simulink model "LQR_EXwithPI"  (Simulink 7.9)
settings: Solver=ode45  StartTime=0.0  StopTime=5  MaxStep=1e-3  RelTol=1e-3
values from neighbouring files (symbols this model uses):
  K1 = K(1,1)    [file_for_LQR_EX.m]
  K2 = K(1,2)    [file_for_LQR_EX.m]
  Q = [2 1; 1 4]    [Riccati_sol2.m]    (also in file_for_LQR_EX.m = [100 0 ; 0 0]; inf_horiz.m = [10 0; 0 2000])
  R = 1/2    (= 0.5)    [Riccati_sol2.m]    (also in file_for_LQR_EX.m = 10; inf_horiz.m = 1)
libraries: simulink x1
settings Model: Creator=DR_C  LastModifiedBy=DR_C
settings DataIOCC: SignalLoggingName=sigsOut
settings OptimizationCC: InitFltsAndDblsToZero=on
settings DebuggingCC: SaveWithParameterizedLinksMsg=none  SignalResolutionControl=TryResolveAllWithWarning  SolverPrmCheckMsg=none  MultiTaskDSMMsg=warning  MultiTaskCondExecSysMsg=none  FcnCallInpInsideContextMsg=Use local settings  StrictBusMsg=Warning
settings HardwareCC: TargetUnknown=on
settings RTWCC: IncludeERTFirstTime=on
settings GRTTargetCC: TargetFcnLib=ansi_tfl_tmw.mat  CombineOutputUpdateFcns=off  GRTInterface=on

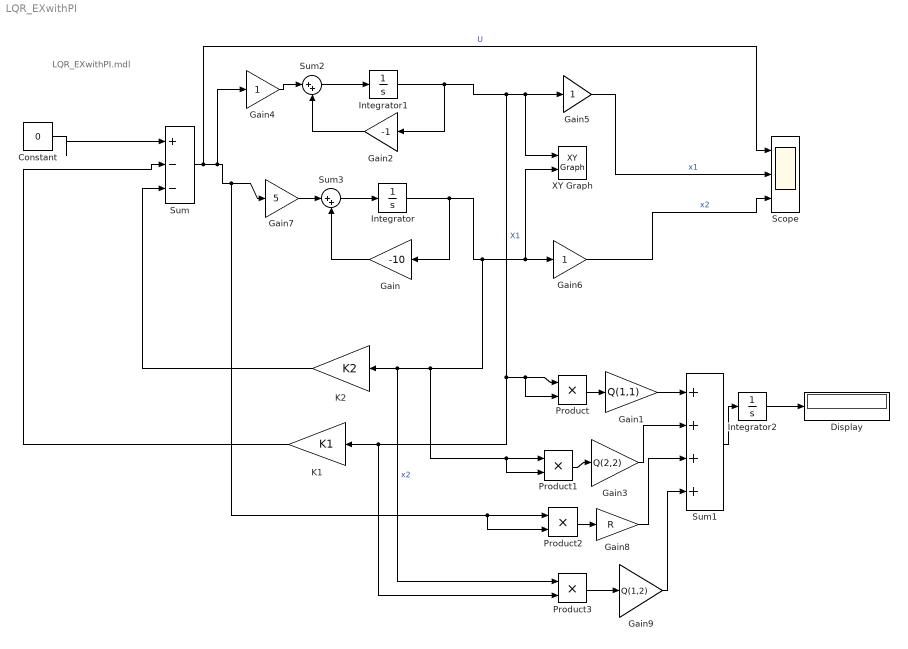
== system LQR_EXwithPI ==
  note: LQR_EXwithPI.mdl
  Constant : Constant  Value=0
  Display : Display
  Gain : Gain  Gain=-10  SaturateOnIntegerOverflow=on  OutDataTypeStr=Inherit: Same as input  ParamDataTypeStr=Inherit: Same as input
  Gain1 : Gain  Gain=Q(1,1)
  Gain2 : Gain  Gain=-1  SaturateOnIntegerOverflow=on  OutDataTypeStr=Inherit: Same as input  ParamDataTypeStr=Inherit: Same as input
  Gain3 : Gain  Gain=Q(2,2)
  Gain4 : Gain  SaturateOnIntegerOverflow=on  OutDataTypeStr=Inherit: Same as input  ParamDataTypeStr=Inherit: Same as input
  Gain5 : Gain  SaturateOnIntegerOverflow=on  OutDataTypeStr=Inherit: Same as input  ParamDataTypeStr=Inherit: Same as input
  Gain6 : Gain  SaturateOnIntegerOverflow=on  OutDataTypeStr=Inherit: Same as input  ParamDataTypeStr=Inherit: Same as input
  Gain7 : Gain  Gain=5  SaturateOnIntegerOverflow=on  OutDataTypeStr=Inherit: Same as input  ParamDataTypeStr=Inherit: Same as input
  Gain8 : Gain  Gain=R
  Gain9 : Gain  Gain=Q(1,2)
  Integrator : Integrator  InitialCondition=10
  Integrator1 : Integrator  InitialCondition=10
  Integrator2 : Integrator
  K1 : Gain  Gain=K1  SaturateOnIntegerOverflow=on  OutDataTypeStr=Inherit: Same as input  ParamDataTypeStr=Inherit: Same as input
  K2 : Gain  Gain=K2  SaturateOnIntegerOverflow=on  OutDataTypeStr=Inherit: Same as input  ParamDataTypeStr=Inherit: Same as input
  Product{,1..3} (4 alike) : Product  RndMeth=Zero
  Scope : Scope  NumInputPorts=3
      settings: YMin=-0.009~0~-0.007  YMax=0~0.004~0
  Sum : Sum  Inputs=|+--  SaturateOnIntegerOverflow=on
  Sum1 : Sum  Inputs=++++
  Sum2 : Sum  Inputs=|++  SaturateOnIntegerOverflow=on
  Sum3 : Sum  Inputs=|++  SaturateOnIntegerOverflow=on
  XY Graph : simulink/Sinks/XY Graph  xmin=-10  xmax=10  ymin=-10  ymax=10  st=-1
  wires:
  Gain5/1 -> Scope/2  "x1"
  Gain6/1 -> Scope/3  "x2"
  Integrator1/1 -> Gain2/1, Gain5/1, XY Graph/1, Product/1, Product/2, K1/1, Product3/2  "X1"
  Integrator/1 -> Gain/1, Gain6/1, XY Graph/2, Product1/1, Product1/2, K2/1, Product3/1  "x2"
  Sum/1 -> Gain4/1, Gain7/1, Product2/1, Product2/2, Scope/1  "U"
  K1/1 -> Sum/2
  Sum3/1 -> Integrator/1
  Gain/1 -> Sum3/2
  Sum2/1 -> Integrator1/1
  Gain2/1 -> Sum2/2
  Gain7/1 -> Sum3/1
  Gain4/1 -> Sum2/1
  K2/1 -> Sum/3
  Constant/1 -> Sum/1
  Integrator2/1 -> Display/1
  Sum1/1 -> Integrator2/1
  Gain1/1 -> Sum1/1
  Product/1 -> Gain1/1
  Product1/1 -> Gain3/1
  Gain3/1 -> Sum1/2
  Product2/1 -> Gain8/1
  Gain8/1 -> Sum1/3
  Product3/1 -> Gain9/1
  Gain9/1 -> Sum1/4
